simulink model "wlan_phy_tx_pmd"  (Simulink 7.8)
settings: Solver=VariableStepDiscrete  SolverMode=SingleTasking  StartTime=0.0  StopTime=inf  RelTol=1e-3
PostLoadFcn:
  | wlan_phy_tx_init
InitFcn:
  | wlan_phy_tx_init
StartFcn:
  | wlan_phy_tx_init
undefined symbols (not defined in the file): gcbh, ht_preamble_rom, MAX_CP_LEN, MAX_DATA_BITS_PER_SYM_PERIOD, MAX_NCBPS, MAX_NUM_BYTES, MAX_NUM_SC, MAX_NUM_SYMS, mcs_rom_11ag, mcs_rom_11n, Mod_Constellation_16QAM, Mod_Constellation_64QAM, Mod_Constellation_BPSK, Mod_Constellation_QPSK, Preamble_IQ, Preamble_IQ_scaled, tx_sim, wlan_tx_interleave_rom, xlBlockLoadCallback, xlGetNormalizedPeriod
libraries: xbsIndex_r4 x1358, xbsEDKLib_r4 x1
(part 4 of 10)

== system wlan_phy_tx_pmd/IFFT and Cyclic Prefix/Buffer and Cyclic Prefix ==
  note: TODO: Use Sym Cfg values for Cyclic Prefix
      | and Cyclic Shift. Will require buffering through
      | FFT somehow, to keep cfg aligned with corresponding
      | samples. Can't assume upstream logic wil hold cfg
      | constant for duration of IFFT processing...
  I : Inport
  Q : Inport  Port=2
  xkindex : Inport  Port=3
  tvalid : Inport  Port=4
  tlast : Inport  Port=5
  Sym Cfg : Inport  Port=6
  AddSub1 : xbsIndex_r4/AddSub  mode=Addition  use_carryin=off  use_carryout=off  en=off  latency=0  precision=User Defined  arith_type=Unsigned  n_bits=ceil(log2(MAX_NUM_SC))  bin_pt=0  quantization=Truncate  overflow=Wrap  dbl_ovrd=off  use_behavioral_HDL=off  hw_selection=Fabric  pipelined=off  block_type=addsub
  AddSub2 : xbsIndex_r4/AddSub  mode=Subtraction  use_carryin=off  use_carryout=off  en=off  latency=1  precision=Full  arith_type=Unsigned  n_bits=MAX_NUM_SC  bin_pt=14  quantization=Truncate  overflow=Wrap  dbl_ovrd=off  use_behavioral_HDL=off  hw_selection=Fabric  pipelined=off  block_type=addsub
  Constant1 : xbsIndex_r4/Constant  const=0  gui_display_data_type=Fixed-point  arith_type=Unsigned  n_bits=32  bin_pt=0  preci_type=Single  exp_width=8  frac_width=24  explicit_period=off  period=1  equ=P=C  opselect=C  inp2=PCIN>>17  opr=+  inp1=P  carry=CIN  dbl_ovrd=off  block_type=constant
      settings: block_version=VER_STRING_GOES_HERE
  Constant2 : xbsIndex_r4/Constant  const=0  gui_display_data_type=Boolean  arith_type=Boolean  n_bits=1  bin_pt=0  preci_type=Single  exp_width=8  frac_width=24  explicit_period=off  period=1  equ=P=C  opselect=C  inp2=PCIN>>17  opr=+  inp1=P  carry=CIN  dbl_ovrd=off  block_type=constant
      settings: block_version=VER_STRING_GOES_HERE
  Control : Subsystem
  Delay : xbsIndex_r4/Delay  rst=off  infoeditControl=Selection of Reset will increase slice count due to use of real FFs and instead of SRLs  en=off  latency=1  dbl_ovrd=off  reg_retiming=off  block_type=delay
  Delay3 : xbsIndex_r4/Delay  rst=off  infoeditControl=Selection of Reset will increase slice count due to use of real FFs and instead of SRLs  en=off  latency=1  dbl_ovrd=off  reg_retiming=off  block_type=delay
  Dual Port RAM : xbsIndex_r4/Dual Port RAM  depth=MAX_NUM_SC * 1  initVector=0  distributed_mem=Block RAM  init_a=0  init_b=0  rst_a=off  rst_b=off  en_a=off  en_b=off  latency=1  write_mode_A=Read After Write  write_mode_B=Read After Write  dbl_ovrd=off  optimize=Area  block_type=dpram
  Gateway Out{1..8} (8 alike) : xbsIndex_r4/Gateway Out  inherit_from_input=off  hdl_port=off  timing_constraint=None  locs_specified=off  LOCs={}  UseAsDAC=off  DACChannel='1'  block_type=gatewayout
  I/Q Concat : Subsystem
  I/Q Slice : Subsystem
  IFFT Buffer : Scope  NumInputPorts=8
      settings: TimeRange=12000  YMin=0~0~0~0~0~-0.5~-0.5~0  YMax=1~100~1~100~1~0.5~0.5~100
  Terminator : Terminator
  " I" : Outport
  " Q" : Outport  Port=2
  " valid" : Outport  Port=3
  wires:
  I/Q Concat/1(IQ) -> Dual Port RAM/2
  Dual Port RAM/2 -> I/Q Slice/1(IQ)
  I/1 -> I/Q Concat/1(I)
  Q/1 -> I/Q Concat/2(Q)
  xkindex/1 -> Dual Port RAM/1, Gateway Out2/1
  tvalid/1 -> Dual Port RAM/3, Gateway Out1/1
  tlast/1 -> Gateway Out3/1, Control/1(tlast)
  AddSub1/1 -> Dual Port RAM/4, Gateway Out4/1, Delay/1
  [regTx_NUM_SC] -> AddSub2/1
  [regTx_CP_LEN] -> AddSub2/2
  AddSub2/1 -> AddSub1/1
  Constant1/1 -> Dual Port RAM/5
  Constant2/1 -> Dual Port RAM/6
  Dual Port RAM/1 -> Terminator/1
  I/Q Slice/1(I) -> " I"/1, Gateway Out6/1
  I/Q Slice/2(Q) -> " Q"/1, Gateway Out8/1
  Gateway Out1/1 -> IFFT Buffer/1  "IN tvalid"
  Gateway Out2/1 -> IFFT Buffer/2  "IN xkindex"
  Gateway Out3/1 -> IFFT Buffer/3  "IN tlast"
  Gateway Out4/1 -> IFFT Buffer/4  "Rd Addr"
  Gateway Out5/1 -> IFFT Buffer/5  "OUT valid"
  Gateway Out6/1 -> IFFT Buffer/6  "OUT I"
  Gateway Out7/1 -> IFFT Buffer/8  "OUT index"
  Control/2(Valid) -> Delay3/1
  Gateway Out8/1 -> IFFT Buffer/7  "OUT Q"
  Delay/1 -> Gateway Out7/1
  Delay3/1 -> " valid"/1, Gateway Out5/1
  Control/1(Rd Addr) -> AddSub1/2
  Sym Cfg/1 -> ?

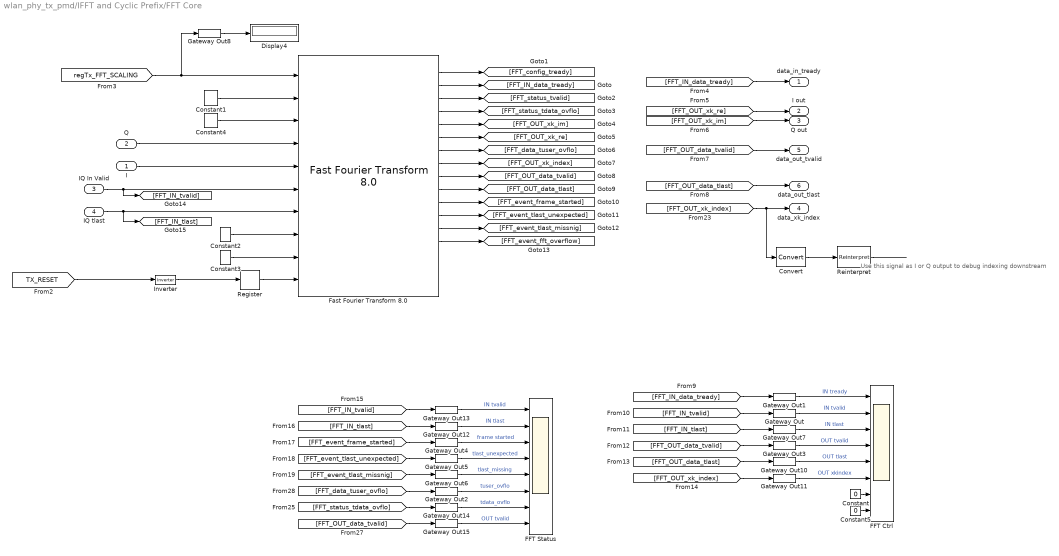
== system wlan_phy_tx_pmd/IFFT and Cyclic Prefix/FFT Core ==
  note: Use this signal as I or Q output
      | to debug indexing downstream
  "I " : Inport
  "Q " : Inport  Port=2
  IQ In Valid : Inport  Port=3
  IQ tlast : Inport  Port=4
  Constant : Constant  Value=0
  Constant1 : xbsIndex_r4/Constant  const=0  gui_display_data_type=Fixed-point  arith_type=Unsigned  n_bits=1  bin_pt=0  preci_type=Single  exp_width=8  frac_width=24  explicit_period=on  period=1  equ=P=C  opselect=C  inp2=PCIN>>17  opr=+  inp1=P  carry=CIN  dbl_ovrd=off  block_type=constant
  Constant2 : xbsIndex_r4/Constant  const=1  gui_display_data_type=Boolean  arith_type=Boolean  n_bits=1  bin_pt=0  preci_type=Single  exp_width=8  frac_width=24  explicit_period=on  period=1  equ=P=C  opselect=C  inp2=PCIN>>17  opr=+  inp1=P  carry=CIN  dbl_ovrd=off  block_type=constant
  Constant3 : xbsIndex_r4/Constant  const=1  gui_display_data_type=Boolean  arith_type=Boolean  n_bits=1  bin_pt=0  preci_type=Single  exp_width=8  frac_width=24  explicit_period=on  period=1  equ=P=C  opselect=C  inp2=PCIN>>17  opr=+  inp1=P  carry=CIN  dbl_ovrd=off  block_type=constant
  Constant4 : xbsIndex_r4/Constant  const=1  gui_display_data_type=Boolean  arith_type=Boolean  n_bits=1  bin_pt=0  preci_type=Single  exp_width=8  frac_width=24  explicit_period=on  period=1  equ=P=C  opselect=C  inp2=PCIN>>17  opr=+  inp1=P  carry=CIN  dbl_ovrd=off  block_type=constant
  Constant5 : Constant  Value=0
  Convert : xbsIndex_r4/Convert  gui_display_data_type=Fixed-point  arith_type="Signed  (2's comp)"  n_bits=16  bin_pt=0  float_type=Single  exp_bits=8  fraction_bits=24  quantization=Truncate  overflow=Wrap  en=off  latency=0  dbl_ovrd=off  pipeline=off  block_type=convert
  Display4 : Display
  FFT Ctrl : Scope  NumInputPorts=8
      settings: TimeRange=4500  YMin=0~0~0~0~0~0~-1~-1  YMax=1~1~1~1~1~80~1~1  SaveName=ScopeData12
  FFT Status : Scope  NumInputPorts=8
      settings: TimeRange=10000  YMin=0~0~0~-1~-1~0~0~0  YMax=1~1~1~1~1~6~6~1  SaveName=ScopeData13
  "Fast Fourier Transform 8.0 " : xbsIndex_r4/Fast Fourier Transform 8.0   transform_length=64  target_clock_frequency=160  target_data_throughput=50  implementation_options=radix_4_burst_io  run_time_configurable_transform_length=off  phase_factor_width=16  scaling_options=scaled  rounding_modes=truncation  aclken=off  aresetn=on  cyclic_prefix_insertion=off  output_ordering=bit_reversed_order  throttle_scheme=nonrealtime  xk_index=on  ovflo=on  trim_axipin_name=on  memory_options_data=block_ram  memory_options_phase_factors=block_ram  number_of_stages_using_block_ram_for_data_and_phase_factors=0  memory_options_reorder=block_ram  memory_options_hybrid=off  complex_mult_type=use_mults_performance  butterfly_type=use_xtremedsp_slices  channels=1  input_ordering=natural_order  input_width=16  ip_name=Fast Fourier Transform  ip_version=8.0  dsptool_ready=true  ipcore_usecache=true  ipcore_useipmodelcache=true  wrapper_available=true  port_translation_map={ 'aclken' => 'en', 'aresetn' => 'rst'}  block_type=xfft_v8_0
  Gateway Out{,1..8,10..15} (15 alike) : xbsIndex_r4/Gateway Out  inherit_from_input=off  hdl_port=off  timing_constraint=None  locs_specified=off  LOCs={}  UseAsDAC=off  DACChannel='1'  block_type=gatewayout
  Inverter : xbsIndex_r4/Inverter  en=off  latency=0  dbl_ovrd=off  block_type=inv
  Register : xbsIndex_r4/Register  init=0  rst=off  en=off  dbl_ovrd=off  block_type=register
  Reinterpret : xbsIndex_r4/Reinterpret  force_arith_type=on  arith_type="Signed  (2's comp)"  force_bin_pt=on  bin_pt=15  block_type=reinterpret
  data_in_tready : Outport
  I out : Outport  Port=2
  Q out : Outport  Port=3
  data_xk_index : Outport  Port=4
  data_out_tvalid : Outport  Port=5
  data_out_tlast : Outport  Port=6
  wires:
  Gateway Out8/1 -> Display4/1
  [regTx_FFT_SCALING] -> Gateway Out8/1, "Fast Fourier Transform 8.0 "/1
  [TX_RESET] -> Inverter/1
  IQ In Valid/1 -> [FFT_IN_tvalid], "Fast Fourier Transform 8.0 "/6
  IQ tlast/1 -> [FFT_IN_tlast], "Fast Fourier Transform 8.0 "/7
  Gateway Out7/1 -> FFT Ctrl/3  "IN tlast"
  Gateway Out6/1 -> FFT Status/5  "tlast_missing"
  Gateway Out5/1 -> FFT Status/4  "tlast_unexpected"
  Gateway Out4/1 -> FFT Status/3  "frame started"
  Gateway Out1/1 -> FFT Ctrl/1  "IN tready"
  Gateway Out/1 -> FFT Ctrl/2  "IN tvalid"
  [FFT_IN_data_tready] -> data_in_tready/1
  [FFT_OUT_xk_re] -> I out/1
  [FFT_OUT_xk_im] -> Q out/1
  [FFT_OUT_data_tvalid] -> data_out_tvalid/1
  [FFT_OUT_data_tlast] -> data_out_tlast/1
  Gateway Out3/1 -> FFT Ctrl/4  "OUT tvalid"
  Gateway Out10/1 -> FFT Ctrl/5  "OUT tlast"
  Gateway Out11/1 -> FFT Ctrl/6  "OUT xkindex"
  Gateway Out12/1 -> FFT Status/2  "IN tlast"
  Gateway Out13/1 -> FFT Status/1  "IN tvalid"
  [FFT_IN_data_tready] -> Gateway Out1/1
  [FFT_IN_tvalid] -> Gateway Out/1
  [FFT_IN_tlast] -> Gateway Out7/1
  [FFT_OUT_data_tvalid] -> Gateway Out3/1
  [FFT_OUT_data_tlast] -> Gateway Out10/1
  [FFT_OUT_xk_index] -> Gateway Out11/1
  [FFT_IN_tvalid] -> Gateway Out13/1
  [FFT_IN_tlast] -> Gateway Out12/1
  [FFT_event_frame_started] -> Gateway Out4/1
  [FFT_event_tlast_unexpected] -> Gateway Out5/1
  [FFT_event_tlast_missnig] -> Gateway Out6/1
  [FFT_OUT_xk_index] -> data_xk_index/1, Convert/1
  Constant/1 -> FFT Ctrl/7
  Constant5/1 -> FFT Ctrl/8
  Gateway Out15/1 -> FFT Status/8  "OUT tvalid"
  [FFT_OUT_data_tvalid] -> Gateway Out15/1
  Constant1/1 -> "Fast Fourier Transform 8.0 "/2
  Constant4/1 -> "Fast Fourier Transform 8.0 "/3
  "Q "/1 -> "Fast Fourier Transform 8.0 "/4
  "I "/1 -> "Fast Fourier Transform 8.0 "/5
  Constant2/1 -> "Fast Fourier Transform 8.0 "/8
  Inverter/1 -> Register/1
  Constant3/1 -> "Fast Fourier Transform 8.0 "/9
  [FFT_data_tuser_ovflo] -> Gateway Out2/1
  Gateway Out2/1 -> FFT Status/6  "tuser_ovflo"
  Gateway Out14/1 -> FFT Status/7  "tdata_ovflo"
  [FFT_status_tdata_ovflo] -> Gateway Out14/1
  "Fast Fourier Transform 8.0 "/1 -> [FFT_config_tready]
  "Fast Fourier Transform 8.0 "/2 -> [FFT_IN_data_tready]
  "Fast Fourier Transform 8.0 "/3 -> [FFT_status_tvalid]
  "Fast Fourier Transform 8.0 "/4 -> [FFT_status_tdata_ovflo]
  "Fast Fourier Transform 8.0 "/5 -> [FFT_OUT_xk_im]
  "Fast Fourier Transform 8.0 "/6 -> [FFT_OUT_xk_re]
  "Fast Fourier Transform 8.0 "/7 -> [FFT_data_tuser_ovflo]
  "Fast Fourier Transform 8.0 "/8 -> [FFT_OUT_xk_index]
  "Fast Fourier Transform 8.0 "/9 -> [FFT_OUT_data_tvalid]
  "Fast Fourier Transform 8.0 "/10 -> [FFT_OUT_data_tlast]
  "Fast Fourier Transform 8.0 "/11 -> [FFT_event_frame_started]
  "Fast Fourier Transform 8.0 "/12 -> [FFT_event_tlast_unexpected]
  "Fast Fourier Transform 8.0 "/13 -> [FFT_event_tlast_missnig]
  "Fast Fourier Transform 8.0 "/14 -> [FFT_event_fft_overflow]
  Convert/1 -> Reinterpret/1
  Reinterpret/1 -> ?
  Register/1 -> "Fast Fourier Transform 8.0 "/10

== system wlan_phy_tx_pmd/IFFT and Cyclic Prefix/FIFO ==
  note: AND not strictly necessary, since FFT
      | only honors tlast when tvalid is asserted.
      | Explicit AND here makes scopes
      | much easier to understand.
  note: This FIFO aids in synchronizing sample generation
      | and feeding the FFT. It would be possible to design
      | the sample buffer control logic not to require
      | this FIFO, but then the logic would need tweaking
      | if the FFT timing or sample processing timing
      | ever change. This FIFO isolates those blocks,
      | at the cost of a little memory
  FFT tready : Inport
  Sym Cfg : Inport  Port=2
  I : Inport  Port=3
  Q : Inport  Port=4
  IQ tvalid : Inport  Port=5
  "IQ tlast " : Inport  Port=6
  AXI FIFO : xbsIndex_r4/AXI FIFO  input_depth_axis=128  actual_fifo_depth_label=130  enable_tdata=on  enable_tdest=off  enable_tstrb=off  enable_tready=on  enable_tid=off  enable_tuser=on  enable_tkeep=off  enable_tlast=on  has_aresetn=on  enable_data_counts_axis=on  fifo_implementation_type_axis=Common Clock Block RAM  trim_axipin_name=on  programmable_full_type_axis=Full  full_threshold_assert_value_axis=0  programmable_empty_type_axis=Empty  empty_threshold_assert_value_axis=1022  block_type=axi_fifo
  Convert : xbsIndex_r4/Convert  gui_display_data_type=Fixed-point  arith_type="Signed  (2's comp)"  n_bits=16  bin_pt=15  float_type=Single  exp_bits=8  fraction_bits=24  quantization=Truncate  overflow=Wrap  en=off  latency=0  dbl_ovrd=off  pipeline=off  block_type=convert
  Convert1 : xbsIndex_r4/Convert  gui_display_data_type=Fixed-point  arith_type="Signed  (2's comp)"  n_bits=16  bin_pt=15  float_type=Single  exp_bits=8  fraction_bits=24  quantization=Truncate  overflow=Wrap  en=off  latency=0  dbl_ovrd=off  pipeline=off  block_type=convert
  FFT IN FIFO : Scope  NumInputPorts=7
      settings: TimeRange=30000  YMin=0~0~0~-0.1~0~-0.1~-0.1  YMax=300~300~1~1.1~4000~1.1~1.1  SaveName=ScopeData20
  FIFO Ctrl : Scope  NumInputPorts=8
      settings: TimeRange=12000  YMin=0~0~0~0~0~0~0~-5  YMax=1~1~5000~1~1~5000~1~5  SaveName=ScopeData21
  Gateway Out{1..15} (15 alike) : xbsIndex_r4/Gateway Out  inherit_from_input=off  hdl_port=off  timing_constraint=None  locs_specified=off  LOCs={}  UseAsDAC=off  DACChannel='1'  block_type=gatewayout
  I/Q Concat : Subsystem
  I/Q Slice : Subsystem
  Inverter : xbsIndex_r4/Inverter  en=off  latency=0  dbl_ovrd=off  block_type=inv
  Logical2 : xbsIndex_r4/Logical  logical_function=AND  inputs=2  en=off  latency=0  precision=Full  arith_type=Unsigned  n_bits=16  bin_pt=0  align_bp=on  dbl_ovrd=off  block_type=logical
  Register : xbsIndex_r4/Register  init=0  rst=off  en=off  dbl_ovrd=off  block_type=register
  " I" : Outport
  " Q" : Outport  Port=2
  " IQ tvalid" : Outport  Port=3
  IQ tlast : Outport  Port=4
  Sym cfg : Outport  Port=5
  FIFO tready : Outport  Port=6
  tag scope: IFFT_FIFO_OCC=global
  wires:
  FFT tready/1 -> Gateway Out8/1, AXI FIFO/2
  IQ tvalid/1 -> AXI FIFO/3, Gateway Out5/1, Gateway Out14/1
  "IQ tlast "/1 -> AXI FIFO/5, Gateway Out6/1, Gateway Out7/1
  I/1 -> Convert/1
  Q/1 -> Convert1/1
  I/Q Concat/1(IQ) -> AXI FIFO/4
  [TX_RESET] -> Inverter/1, Gateway Out13/1
  Inverter/1 -> Register/1
  Convert/1 -> I/Q Concat/1(I)
  Convert1/1 -> I/Q Concat/2(Q)
  Sym Cfg/1 -> AXI FIFO/6, Gateway Out9/1
  AXI FIFO/5 -> FIFO tready/1, Gateway Out4/1
  AXI FIFO/2 -> I/Q Slice/1(IQ)
  AXI FIFO/1 -> " IQ tvalid"/1, Gateway Out1/1, Logical2/1, Gateway Out10/1
  AXI FIFO/3 -> Logical2/2, Gateway Out11/1
  Gateway Out8/1 -> FFT IN FIFO/1  "FFT ready"
  I/Q Slice/1(I) -> " I"/1
  I/Q Slice/2(Q) -> " Q"/1, Gateway Out2/1
  Gateway Out1/1 -> FFT IN FIFO/2  "FIFO out valid"
  Gateway Out2/1 -> FFT IN FIFO/3  "Q out"
  Gateway Out3/1 -> FFT IN FIFO/4  "tlast out"
  Gateway Out4/1 -> FFT IN FIFO/5  "FIFO ready"
  Gateway Out5/1 -> FFT IN FIFO/6  "valid in"
  Gateway Out6/1 -> FFT IN FIFO/7  "tlast in"
  Logical2/1 -> IQ tlast/1, Gateway Out3/1
  AXI FIFO/4 -> Gateway Out12/1, Sym cfg/1
  Gateway Out14/1 -> FIFO Ctrl/1  "VALID In"
  Gateway Out7/1 -> FIFO Ctrl/2  "TLAST In"
  Gateway Out9/1 -> FIFO Ctrl/3  "TUSER In"
  Gateway Out10/1 -> FIFO Ctrl/4  "VALID out"
  Gateway Out11/1 -> FIFO Ctrl/5  "TLAST out"
  Gateway Out12/1 -> FIFO Ctrl/6  "TUSER out"
  Gateway Out13/1 -> FIFO Ctrl/7  "Reset"
  AXI FIFO/6 -> [IFFT_FIFO_OCC], Gateway Out15/1
  Register/1 -> AXI FIFO/1
  Gateway Out15/1 -> FIFO Ctrl/8  "FIFO Occ"

== system wlan_phy_tx_pmd/OFDM Symbol Ctrl/Posedge1 ==
  D : Inport
  Delay : xbsIndex_r4/Delay  rst=off  infoeditControl=Selection of Reset will increase slice count due to use of real FFs and instead of SRLs  en=off  latency=1  dbl_ovrd=off  reg_retiming=off  block_type=delay
      settings: infoedit=Hardware notes: A delay line is a chain, each link of which is an SRL16 followed by a flip-flop. If register retiming is enabled, the delay line is a chain of flip-flops.  xl_area=[1 1 0 0 0 0 0]  block_version=VER_STRING_GOES_HERE
  Inverter : xbsIndex_r4/Inverter  en=off  latency=0  dbl_ovrd=off  block_type=inv
      settings: xl_area=[0 0 0 0 0 0 0]  block_version=VER_STRING_GOES_HERE
  Logical1 : xbsIndex_r4/Logical  logical_function=AND  inputs=2  en=off  latency=0  precision=Full  arith_type=Unsigned  n_bits=8  bin_pt=2  align_bp=on  dbl_ovrd=off  block_type=logical
      settings: xl_area=[1 0 0 1 0 0 0]  block_version=VER_STRING_GOES_HERE
  Q : Outport
  wires:
  Inverter/1 -> Logical1/1
  D/1 -> Logical1/2, Delay/1
  Logical1/1 -> Q/1
  Delay/1 -> Inverter/1

== system wlan_phy_tx_pmd/OFDM Symbol Ctrl/Posedge2 ==
  D : Inport
  Delay : xbsIndex_r4/Delay  rst=off  infoeditControl=Selection of Reset will increase slice count due to use of real FFs and instead of SRLs  en=off  latency=1  dbl_ovrd=off  reg_retiming=off  block_type=delay
      settings: infoedit=Hardware notes: A delay line is a chain, each link of which is an SRL16 followed by a flip-flop. If register retiming is enabled, the delay line is a chain of flip-flops.  xl_area=[1 1 0 0 0 0 0]  block_version=VER_STRING_GOES_HERE
  Inverter : xbsIndex_r4/Inverter  en=off  latency=0  dbl_ovrd=off  block_type=inv
      settings: xl_area=[0 0 0 0 0 0 0]  block_version=VER_STRING_GOES_HERE
  Logical1 : xbsIndex_r4/Logical  logical_function=AND  inputs=2  en=off  latency=0  precision=Full  arith_type=Unsigned  n_bits=8  bin_pt=2  align_bp=on  dbl_ovrd=off  block_type=logical
      settings: xl_area=[1 0 0 1 0 0 0]  block_version=VER_STRING_GOES_HERE
  Q : Outport
  wires:
  Delay/1 -> Inverter/1
  Logical1/1 -> Q/1
  D/1 -> Delay/1, Logical1/2
  Inverter/1 -> Logical1/1

== system wlan_phy_tx_pmd/OFDM Symbol Ctrl/Posedge3 ==
  D : Inport
  Delay : xbsIndex_r4/Delay  rst=off  infoeditControl=Selection of Reset will increase slice count due to use of real FFs and instead of SRLs  en=off  latency=1  dbl_ovrd=off  reg_retiming=off  block_type=delay
      settings: infoedit=Hardware notes: A delay line is a chain, each link of which is an SRL16 followed by a flip-flop. If register retiming is enabled, the delay line is a chain of flip-flops.  xl_area=[1 1 0 0 0 0 0]  block_version=VER_STRING_GOES_HERE
  Inverter : xbsIndex_r4/Inverter  en=off  latency=0  dbl_ovrd=off  block_type=inv
      settings: xl_area=[0 0 0 0 0 0 0]  block_version=VER_STRING_GOES_HERE
  Logical1 : xbsIndex_r4/Logical  logical_function=AND  inputs=2  en=off  latency=0  precision=Full  arith_type=Unsigned  n_bits=8  bin_pt=2  align_bp=on  dbl_ovrd=off  block_type=logical
      settings: xl_area=[1 0 0 1 0 0 0]  block_version=VER_STRING_GOES_HERE
  Q : Outport
  wires:
  Delay/1 -> Inverter/1
  Logical1/1 -> Q/1
  D/1 -> Delay/1, Logical1/2
  Inverter/1 -> Logical1/1

== system wlan_phy_tx_pmd/OFDM Symbol Ctrl/S-R Latch1 ==
  S : Inport
  R : Inport  Port=2
  Constant1 : xbsIndex_r4/Constant  const=1  gui_display_data_type=Fixed-point  arith_type=Boolean  n_bits=1  bin_pt=0  preci_type=Single  exp_width=8  frac_width=24  explicit_period=off  period=1  equ=P=C  opselect=C  inp2=PCIN>>17  opr=+  inp1=P  carry=CIN  dbl_ovrd=off  block_type=constant
      settings: block_version=VER_STRING_GOES_HERE
  Convert1 : xbsIndex_r4/Convert  gui_display_data_type=Boolean  arith_type=Boolean  n_bits=1  bin_pt=0  float_type=Single  exp_bits=8  fraction_bits=24  quantization=Truncate  overflow=Wrap  en=off  latency=0  dbl_ovrd=off  pipeline=off  block_type=convert
  Convert2 : xbsIndex_r4/Convert  gui_display_data_type=Boolean  arith_type=Boolean  n_bits=1  bin_pt=0  float_type=Single  exp_bits=8  fraction_bits=24  quantization=Truncate  overflow=Wrap  en=off  latency=0  dbl_ovrd=off  pipeline=off  block_type=convert
  Register2 : xbsIndex_r4/Register  init=0  rst=on  en=on  dbl_ovrd=off  block_type=register
      settings: xl_area=[1 1 0 0 0 0 0]  block_version=VER_STRING_GOES_HERE
  Q : Outport
  wires:
  Convert2/1 -> Register2/3
  Convert1/1 -> Register2/2
  Constant1/1 -> Register2/1
  R/1 -> Convert1/1
  Register2/1 -> Q/1
  S/1 -> Convert2/1

== system wlan_phy_tx_pmd/OFDM Symbol Ctrl/S-R Latch2 ==
  S : Inport
  R : Inport  Port=2
  Constant1 : xbsIndex_r4/Constant  const=1  gui_display_data_type=Fixed-point  arith_type=Boolean  n_bits=1  bin_pt=0  preci_type=Single  exp_width=8  frac_width=24  explicit_period=off  period=1  equ=P=C  opselect=C  inp2=PCIN>>17  opr=+  inp1=P  carry=CIN  dbl_ovrd=off  block_type=constant
      settings: block_version=VER_STRING_GOES_HERE
  Convert1 : xbsIndex_r4/Convert  gui_display_data_type=Boolean  arith_type=Boolean  n_bits=1  bin_pt=0  float_type=Single  exp_bits=8  fraction_bits=24  quantization=Truncate  overflow=Wrap  en=off  latency=0  dbl_ovrd=off  pipeline=off  block_type=convert
  Convert2 : xbsIndex_r4/Convert  gui_display_data_type=Boolean  arith_type=Boolean  n_bits=1  bin_pt=0  float_type=Single  exp_bits=8  fraction_bits=24  quantization=Truncate  overflow=Wrap  en=off  latency=0  dbl_ovrd=off  pipeline=off  block_type=convert
  Register2 : xbsIndex_r4/Register  init=0  rst=on  en=on  dbl_ovrd=off  block_type=register
      settings: xl_area=[1 1 0 0 0 0 0]  block_version=VER_STRING_GOES_HERE
  Q : Outport
  wires:
  S/1 -> Convert2/1
  Register2/1 -> Q/1
  R/1 -> Convert1/1
  Constant1/1 -> Register2/1
  Convert1/1 -> Register2/2
  Convert2/1 -> Register2/3

== system wlan_phy_tx_pmd/OFDM Symbol Ctrl/S-R Latch3 ==
  S : Inport
  R : Inport  Port=2
  Constant1 : xbsIndex_r4/Constant  const=1  gui_display_data_type=Fixed-point  arith_type=Boolean  n_bits=1  bin_pt=0  preci_type=Single  exp_width=8  frac_width=24  explicit_period=off  period=1  equ=P=C  opselect=C  inp2=PCIN>>17  opr=+  inp1=P  carry=CIN  dbl_ovrd=off  block_type=constant
      settings: block_version=VER_STRING_GOES_HERE
  Convert1 : xbsIndex_r4/Convert  gui_display_data_type=Boolean  arith_type=Boolean  n_bits=1  bin_pt=0  float_type=Single  exp_bits=8  fraction_bits=24  quantization=Truncate  overflow=Wrap  en=off  latency=0  dbl_ovrd=off  pipeline=off  block_type=convert
  Convert2 : xbsIndex_r4/Convert  gui_display_data_type=Boolean  arith_type=Boolean  n_bits=1  bin_pt=0  float_type=Single  exp_bits=8  fraction_bits=24  quantization=Truncate  overflow=Wrap  en=off  latency=0  dbl_ovrd=off  pipeline=off  block_type=convert
  Register2 : xbsIndex_r4/Register  init=0  rst=on  en=on  dbl_ovrd=off  block_type=register
      settings: xl_area=[1 1 0 0 0 0 0]  block_version=VER_STRING_GOES_HERE
  Q : Outport
  wires:
  S/1 -> Convert2/1
  Register2/1 -> Q/1
  R/1 -> Convert1/1
  Constant1/1 -> Register2/1
  Convert1/1 -> Register2/2
  Convert2/1 -> Register2/3

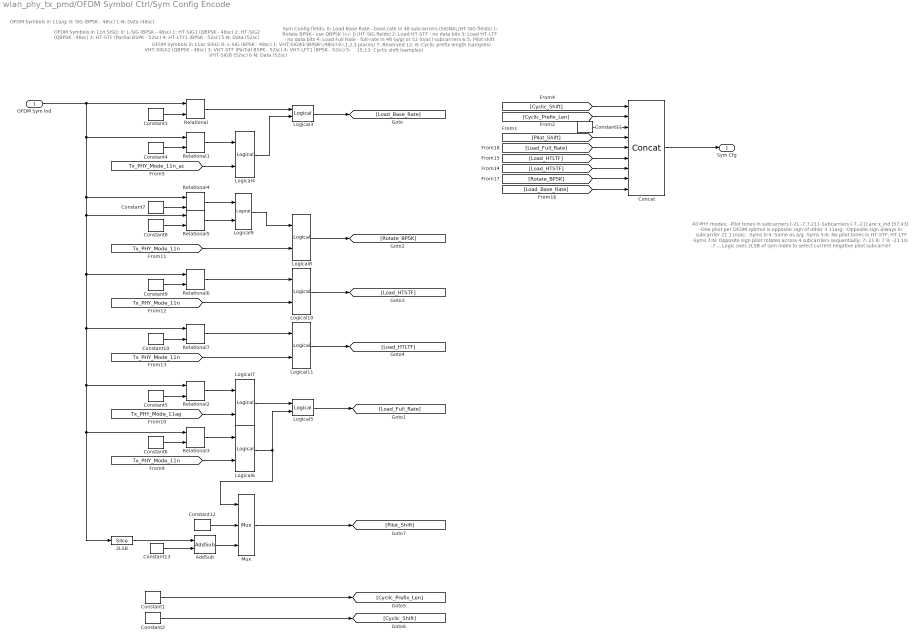
== system wlan_phy_tx_pmd/OFDM Symbol Ctrl/Sym Config Encode ==
  note: Sym Config fields:
      |   0: Load Base Rate - base-rate in 48 subcarriers (SIGNAL/HT-SIG fields)
      |   1: Rotate BPSK - use QBPSK (+/- j) (HT-SIG fields)
      |   2: Load HT-STF - no data bits
      |   3: Load HT-LTF - no data bits
      |   4: Load Full Rate - full-rate in 48 (a/g) or 52 (n/ac) subcarriers
      | 6:5: Pilot shift (Rotate negative pilot 0,1,2,3 places)
      |   7: Reserved
      |
      | 12: 8: Cyclic prefix length (samples)
      | 15:13: Cyclic shift (samples)
  note: OFDM Symbols in 11ac SISO:
      | 0: L-SIG (BPSK - 48sc)
      | 1: VHT-SIGA1 (BPSK - 48sc)
      | 2: VHT-SIGA2 (QBPSK - 48sc)
      | 3: VHT-STF (Partial BSPK - 52sc)
      | 4: VHT-LFT1 (BPSK - 52sc)
      | 5: VHT-SIGB (52sc)
      | 6-N: Data (52sc)
  note: OFDM Symbols in 11n SISO:
      | 0: L-SIG (BPSK - 48sc)
      | 1: HT-SIG1 (QBPSK - 48sc)
      | 2: HT-SIG2 (QBPSK - 48sc)
      | 3: HT-STF (Partial BSPK - 52sc)
      | 4: HT-LTF1 (BPSK - 52sc)
      | 5-N: Data (52sc)
  note: OFDM Symbols in 11a/g:
      | 0: SIG (BPSK - 48sc)
      | 1-N: Data (48sc)
  note: All PHY modes:
      | -Pilot tones in subcarriers [-21,-7,7,21]
      | -Subcarriers [-7,-21] are x_ind [57,43]
      | -One pilot per OFDM sybmol is opposite sign of other 3
      |
      | 11a/g:
      | -Opposite sign always in subcarrier 21
      |
      | 11n/ac:
      | -Syms 0:4: Same as a/g
      | -Syms 5:6: No pilot tones in HT-STF, HT-LTF
      | -Syms 7:N: Opposite sign pilot rotates across 4 subcarriers sequentially:
      |    7: 21
      |    8: 7
      |    9: -21
      |    10: -7
      |     ...
      | Logic uses 2LSB of sym index to select current negative pilot subcarrier
  OFDM Sym Ind : Inport
  2LSB : xbsIndex_r4/Slice  nbits=2  boolean_output=off  mode=Lower Bit Location + Width  bit1=0  base1=MSB of Input  bit0=0  base0=LSB of Input  dbl_ovrd=off  block_type=slice
  AddSub : xbsIndex_r4/AddSub  mode=Addition  use_carryin=off  use_carryout=off  en=off  latency=0  precision=User Defined  arith_type=Unsigned  n_bits=2  bin_pt=0  quantization=Truncate  overflow=Wrap  dbl_ovrd=off  use_behavioral_HDL=off  hw_selection=Fabric  pipelined=off  block_type=addsub
  Concat : xbsIndex_r4/Concat  num_inputs=9  dbl_ovrd=off  block_type=concat
  Constant1 : xbsIndex_r4/Constant  const=16  gui_display_data_type=Fixed-point  arith_type=Unsigned  n_bits=5  bin_pt=0  preci_type=Single  exp_width=8  frac_width=24  explicit_period=on  period=1  equ=P=C  opselect=C  inp2=PCIN>>17  opr=+  inp1=P  carry=CIN  dbl_ovrd=off  block_type=constant
  Constant10 : xbsIndex_r4/Constant  const=4  gui_display_data_type=Fixed-point  arith_type=Unsigned  n_bits=3  bin_pt=0  preci_type=Single  exp_width=8  frac_width=24  explicit_period=off  period=1  equ=P=C  opselect=C  inp2=PCIN>>17  opr=+  inp1=P  carry=CIN  dbl_ovrd=off  block_type=constant
  Constant11 : xbsIndex_r4/Constant  const=0  gui_display_data_type=Fixed-point  arith_type=Unsigned  n_bits=1  bin_pt=0  preci_type=Single  exp_width=8  frac_width=24  explicit_period=off  period=1  equ=P=C  opselect=C  inp2=PCIN>>17  opr=+  inp1=P  carry=CIN  dbl_ovrd=off  block_type=constant
  Constant12 : xbsIndex_r4/Constant  const=0  gui_display_data_type=Fixed-point  arith_type=Unsigned  n_bits=2  bin_pt=0  preci_type=Single  exp_width=8  frac_width=24  explicit_period=off  period=1  equ=P=C  opselect=C  inp2=PCIN>>17  opr=+  inp1=P  carry=CIN  dbl_ovrd=off  block_type=constant
  Constant13 : xbsIndex_r4/Constant  const=3  gui_display_data_type=Fixed-point  arith_type=Unsigned  n_bits=2  bin_pt=0  preci_type=Single  exp_width=8  frac_width=24  explicit_period=off  period=8  equ=P=C  opselect=C  inp2=PCIN>>17  opr=+  inp1=P  carry=CIN  dbl_ovrd=off  block_type=constant
  Constant2 : xbsIndex_r4/Constant  const=0  gui_display_data_type=Fixed-point  arith_type=Unsigned  n_bits=5  bin_pt=0  preci_type=Single  exp_width=8  frac_width=24  explicit_period=on  period=1  equ=P=C  opselect=C  inp2=PCIN>>17  opr=+  inp1=P  carry=CIN  dbl_ovrd=off  block_type=constant
  Constant3 : xbsIndex_r4/Constant  const=0  gui_display_data_type=Fixed-point  arith_type=Unsigned  n_bits=1  bin_pt=0  preci_type=Single  exp_width=8  frac_width=24  explicit_period=off  period=1  equ=P=C  opselect=C  inp2=PCIN>>17  opr=+  inp1=P  carry=CIN  dbl_ovrd=off  block_type=constant
  Constant4 : xbsIndex_r4/Constant  const=2  gui_display_data_type=Fixed-point  arith_type=Unsigned  n_bits=2  bin_pt=0  preci_type=Single  exp_width=8  frac_width=24  explicit_period=off  period=1  equ=P=C  opselect=C  inp2=PCIN>>17  opr=+  inp1=P  carry=CIN  dbl_ovrd=off  block_type=constant
  Constant5 : xbsIndex_r4/Constant  const=1  gui_display_data_type=Fixed-point  arith_type=Unsigned  n_bits=1  bin_pt=0  preci_type=Single  exp_width=8  frac_width=24  explicit_period=off  period=1  equ=P=C  opselect=C  inp2=PCIN>>17  opr=+  inp1=P  carry=CIN  dbl_ovrd=off  block_type=constant
  Constant6 : xbsIndex_r4/Constant  const=5  gui_display_data_type=Fixed-point  arith_type=Unsigned  n_bits=3  bin_pt=0  preci_type=Single  exp_width=8  frac_width=24  explicit_period=off  period=1  equ=P=C  opselect=C  inp2=PCIN>>17  opr=+  inp1=P  carry=CIN  dbl_ovrd=off  block_type=constant
  Constant7 : xbsIndex_r4/Constant  const=1  gui_display_data_type=Fixed-point  arith_type=Unsigned  n_bits=1  bin_pt=0  preci_type=Single  exp_width=8  frac_width=24  explicit_period=off  period=1  equ=P=C  opselect=C  inp2=PCIN>>17  opr=+  inp1=P  carry=CIN  dbl_ovrd=off  block_type=constant
  Constant8 : xbsIndex_r4/Constant  const=2  gui_display_data_type=Fixed-point  arith_type=Unsigned  n_bits=2  bin_pt=0  preci_type=Single  exp_width=8  frac_width=24  explicit_period=off  period=1  equ=P=C  opselect=C  inp2=PCIN>>17  opr=+  inp1=P  carry=CIN  dbl_ovrd=off  block_type=constant
  Constant9 : xbsIndex_r4/Constant  const=3  gui_display_data_type=Fixed-point  arith_type=Unsigned  n_bits=2  bin_pt=0  preci_type=Single  exp_width=8  frac_width=24  explicit_period=off  period=1  equ=P=C  opselect=C  inp2=PCIN>>17  opr=+  inp1=P  carry=CIN  dbl_ovrd=off  block_type=constant
  Logical{4,6..8,10..11} (6 alike) : xbsIndex_r4/Logical  logical_function=AND  inputs=2  en=off  latency=0  precision=Full  arith_type=Unsigned  n_bits=8  bin_pt=2  align_bp=on  dbl_ovrd=off  block_type=logical
      settings: xl_area=[1 0 0 1 0 0 0]  block_version=VER_STRING_GOES_HERE
  Logical3 : xbsIndex_r4/Logical  logical_function=OR  inputs=2  en=off  latency=0  precision=Full  arith_type=Unsigned  n_bits=8  bin_pt=2  align_bp=on  dbl_ovrd=off  block_type=logical
      settings: xl_area=[1 0 0 1 0 0 0]  block_version=VER_STRING_GOES_HERE
  Logical5 : xbsIndex_r4/Logical  logical_function=OR  inputs=2  en=off  latency=0  precision=Full  arith_type=Unsigned  n_bits=8  bin_pt=2  align_bp=on  dbl_ovrd=off  block_type=logical
      settings: xl_area=[1 0 0 1 0 0 0]  block_version=VER_STRING_GOES_HERE
  Logical9 : xbsIndex_r4/Logical  logical_function=OR  inputs=2  en=off  latency=0  precision=Full  arith_type=Unsigned  n_bits=8  bin_pt=2  align_bp=on  dbl_ovrd=off  block_type=logical
      settings: xl_area=[1 0 0 1 0 0 0]  block_version=VER_STRING_GOES_HERE
  Mux : xbsIndex_r4/Mux  inputs=2  en=off  latency=0  precision=Full  arith_type=Unsigned  n_bits=16  bin_pt=14  quantization=Truncate  overflow=Wrap  dbl_ovrd=off  block_type=mux
  Relational{,4..7} (5 alike) : xbsIndex_r4/Relational  mode=a=b  en=off  latency=0  dbl_ovrd=off  block_type=relational
  Relational1 : xbsIndex_r4/Relational  mode=a<=b  en=off  latency=0  dbl_ovrd=off  block_type=relational
  Relational2 : xbsIndex_r4/Relational  mode=a>=b  en=off  latency=0  dbl_ovrd=off  block_type=relational
  Relational3 : xbsIndex_r4/Relational  mode=a>=b  en=off  latency=0  dbl_ovrd=off  block_type=relational
  Sym Cfg : Outport
  wires:
  Constant3/1 -> Relational/2
  Relational/1 -> Logical3/1
  [Tx_PHY_Mode_11n_ac] -> Logical4/2
  Relational1/1 -> Logical4/1
  Constant4/1 -> Relational1/2
  Logical4/1 -> Logical3/2
  Constant5/1 -> Relational2/2
  [Tx_PHY_Mode_11n] -> Logical6/2
  Relational3/1 -> Logical6/1
  Constant6/1 -> Relational3/2
  Logical6/1 -> Logical5/2, Mux/1
  Logical5/1 -> [Load_Full_Rate]
  Logical7/1 -> Logical5/1
  Relational2/1 -> Logical7/1
  [Tx_PHY_Mode_11ag] -> Logical7/2
  [Tx_PHY_Mode_11n] -> Logical8/2
  Constant7/1 -> Relational4/2
  Constant8/1 -> Relational5/2
  Relational4/1 -> Logical9/1
  Relational5/1 -> Logical9/2
  Logical9/1 -> Logical8/1
  Logical8/1 -> [Rotate_BPSK]
  [Tx_PHY_Mode_11n] -> Logical10/2
  Constant9/1 -> Relational6/2
  Relational6/1 -> Logical10/1
  Logical10/1 -> [Load_HTSTF]
  [Tx_PHY_Mode_11n] -> Logical11/2
  Constant10/1 -> Relational7/2
  Relational7/1 -> Logical11/1
  Logical11/1 -> [Load_HTLTF]
  OFDM Sym Ind/1 -> Relational/1, Relational1/1, Relational5/1, Relational6/1, Relational7/1, Relational2/1, Relational3/1, 2LSB/1, Relational4/1
  [Load_Full_Rate] -> Concat/5
  [Load_HTLTF] -> Concat/6
  [Load_HTSTF] -> Concat/7
  [Rotate_BPSK] -> Concat/8
  [Load_Base_Rate] -> Concat/9
  Constant1/1 -> [Cyclic_Prefix_Len]
  Constant2/1 -> [Cyclic_Shift]
  Constant11/1 -> Concat/3
  [Cyclic_Prefix_Len] -> Concat/2
  [Cyclic_Shift] -> Concat/1
  Concat/1 -> Sym Cfg/1
  Logical3/1 -> [Load_Base_Rate]
  2LSB/1 -> AddSub/1
  [Pilot_Shift] -> Concat/4
  Constant12/1 -> Mux/2
  Mux/1 -> [Pilot_Shift]
  AddSub/1 -> Mux/3
  Constant13/1 -> AddSub/2

== system wlan_phy_tx_pmd/OFDM Symbol Ctrl/Sym Counter ==
  note: Use SR latch to skip counter increment
      | on first sym (indexes syms by 0)
  Start Sym : Inport
  Delay : xbsIndex_r4/Delay  rst=off  infoeditControl=Selection of Reset will increase slice count due to use of real FFs and instead of SRLs  en=off  latency=1  dbl_ovrd=off  reg_retiming=off  block_type=delay
  Logical2 : xbsIndex_r4/Logical  logical_function=AND  inputs=2  en=off  latency=0  precision=Full  arith_type=Unsigned  n_bits=8  bin_pt=2  align_bp=on  dbl_ovrd=off  block_type=logical
      settings: xl_area=[1 0 0 1 0 0 0]  block_version=VER_STRING_GOES_HERE
  S-R Latch1 : Subsystem
  Sym Counter : xbsIndex_r4/Counter  cnt_type=Free Running  cnt_to=47  operation=Up  start_count=0  cnt_by_val=1  arith_type=Unsigned  n_bits=ceil(log2(MAX_NUM_SYMS))  bin_pt=0  load_pin=off  rst=on  en=on  explicit_period=off  period=1  dbl_ovrd=off  use_behavioral_HDL=off  implementation=Fabric  block_type=counter
  Sym Ind : Outport
  " Start Sym" : Outport  Port=2
  wires:
  [TX_RESET] -> Sym Counter/1
  Logical2/1 -> Sym Counter/2
  S-R Latch1/1(Q) -> Logical2/2
  [TX_RESET] -> S-R Latch1/2(R)
  Start Sym/1 -> Logical2/1, S-R Latch1/1(S), Delay/1
  Sym Counter/1 -> Sym Ind/1
  Delay/1 -> " Start Sym"/1

== system wlan_phy_tx_pmd/OFDM Symbol Ctrl/Sym Samp Counter ==
  Sym Started : Inport
  Sym Cfg : Inport  Port=2
  AddSub : xbsIndex_r4/AddSub  mode=Addition  use_carryin=off  use_carryout=off  en=on  latency=1  precision=Full  arith_type=Unsigned  n_bits=16  bin_pt=14  quantization=Truncate  overflow=Wrap  dbl_ovrd=off  use_behavioral_HDL=off  hw_selection=Fabric  pipelined=off  block_type=addsub
  Inverter : xbsIndex_r4/Inverter  en=off  latency=0  dbl_ovrd=off  block_type=inv
  Logical : xbsIndex_r4/Logical  logical_function=AND  inputs=2  en=off  latency=0  precision=Full  arith_type=Unsigned  n_bits=16  bin_pt=0  align_bp=on  dbl_ovrd=off  block_type=logical
  Logical1 : xbsIndex_r4/Logical  logical_function=OR  inputs=2  en=off  latency=0  precision=Full  arith_type=Unsigned  n_bits=16  bin_pt=0  align_bp=on  dbl_ovrd=off  block_type=logical
  Logical2 : xbsIndex_r4/Logical  logical_function=OR  inputs=2  en=off  latency=0  precision=Full  arith_type=Unsigned  n_bits=16  bin_pt=0  align_bp=on  dbl_ovrd=off  block_type=logical
  MCode : xbsIndex_r4/MCode  mfname=sym_config_decode  explicit_period=on  period=1  inputsTable={'boundInpExpr'=>[''],'inputs'=>['sym_cfg']}  outputsTable={'outputs'=>['load_base_rate','rotate_bpsk','load_htstf','load_htltf','load_full_rate','pilot_shift','cyclic_prefix','cyclic_shift'],'suppressOut'=>['off','off','off','off','off','off','off','off']}  dbl_ovrd=off  enable_stdout=off  enable_debug=off  suppress_output=on  defparams={}  hide_port_list={}  block_type=mcode
  Posedge1 : Subsystem
  Posedge2 : Subsystem
  Relational2 : xbsIndex_r4/Relational  mode=a>=b  en=off  latency=0  dbl_ovrd=off  block_type=relational
  S-R Latch2 : Subsystem
  Samp Counter : xbsIndex_r4/Counter  cnt_type=Free Running  cnt_to=47  operation=Up  start_count=0  cnt_by_val=1  arith_type=Unsigned  n_bits=ceil(log2(MAX_NUM_SYMS))  bin_pt=0  load_pin=off  rst=on  en=on  explicit_period=off  period=1  dbl_ovrd=off  use_behavioral_HDL=off  implementation=Fabric  block_type=counter
  Start Next : Outport
  wires:
  Logical/1 -> Samp Counter/2
  [regTx_NUM_SC] -> AddSub/1
  Sym Cfg/1 -> MCode/1
  Samp Counter/1 -> Relational2/1
  MCode/7 -> AddSub/2
  Sym Started/1 -> Posedge1/1(D)
  Posedge1/1(Q) -> S-R Latch2/1(S)
  S-R Latch2/1(Q) -> Logical/1, Inverter/1
  [TX_IQ_SAMP_CE] -> Logical/2
  Relational2/1 -> Posedge2/1(D)
  AddSub/1 -> Relational2/2
  Posedge2/1(Q) -> Start Next/1, Logical1/2
  Logical1/1 -> S-R Latch2/2(R)
  Logical2/1 -> Samp Counter/1
  Inverter/1 -> Logical2/2
  [TX_RESET] -> Logical2/1, Logical1/1, AddSub/3

== system wlan_phy_tx_pmd/PSDU Syms Gen/Convolutional Encoder ==
  Sym Cfg : Inport
  Tx Bit : Inport  Port=2
  Tx Bit tvalid : Inport  Port=3
  Tx Bit tlast : Inport  Port=4
  A XOR : xbsIndex_r4/Logical  logical_function=XOR  inputs=5  en=on  latency=1  precision=Full  arith_type=Unsigned  n_bits=8  bin_pt=2  align_bp=on  dbl_ovrd=off  block_type=logical
      settings: xl_area=[0, 0, 0, 0, 0, 0, 0]  block_version=VER_STRING_GOES_HERE
  B XOR : xbsIndex_r4/Logical  logical_function=XOR  inputs=5  en=on  latency=1  precision=Full  arith_type=Unsigned  n_bits=8  bin_pt=2  align_bp=on  dbl_ovrd=off  block_type=logical
      settings: xl_area=[0, 0, 0, 0, 0, 0, 0]  block_version=VER_STRING_GOES_HERE
  Concat : xbsIndex_r4/Concat  num_inputs=2  dbl_ovrd=off  block_type=concat
  Convert : xbsIndex_r4/Convert  gui_display_data_type=Boolean  arith_type=Boolean  n_bits=16  bin_pt=14  float_type=Single  exp_bits=8  fraction_bits=24  quantization=Truncate  overflow=Wrap  en=off  latency=0  dbl_ovrd=off  pipeline=off  block_type=convert
  Convert2 : xbsIndex_r4/Convert  gui_display_data_type=Boolean  arith_type=Boolean  n_bits=16  bin_pt=14  float_type=Single  exp_bits=8  fraction_bits=24  quantization=Truncate  overflow=Wrap  en=off  latency=0  dbl_ovrd=off  pipeline=off  block_type=convert
  Delay1 : xbsIndex_r4/Delay  rst=off  infoeditControl=Selection of Reset will increase slice count due to use of real FFs and instead of SRLs  en=off  latency=1  dbl_ovrd=off  reg_retiming=off  block_type=delay
  Delay2 : xbsIndex_r4/Delay  rst=off  infoeditControl=Selection of Reset will increase slice count due to use of real FFs and instead of SRLs  en=off  latency=1  dbl_ovrd=off  reg_retiming=off  block_type=delay
  Delay3 : xbsIndex_r4/Delay  rst=off  infoeditControl=Selection of Reset will increase slice count due to use of real FFs and instead of SRLs  en=off  latency=1  dbl_ovrd=off  reg_retiming=off  block_type=delay
  Gateway Out1 : xbsIndex_r4/Gateway Out  inherit_from_input=off  hdl_port=off  timing_constraint=None  locs_specified=off  LOCs={}  UseAsDAC=off  DACChannel='1'  block_type=gatewayout
  Gateway Out4 : xbsIndex_r4/Gateway Out  inherit_from_input=off  hdl_port=off  timing_constraint=None  locs_specified=off  LOCs={}  UseAsDAC=off  DACChannel='1'  block_type=gatewayout
  Register{,1..5} (6 alike) : xbsIndex_r4/Register  init=0  rst=on  en=on  dbl_ovrd=off  block_type=register
      settings: xl_area=[0, 0, 0, 0, 0, 0, 0]  block_version=VER_STRING_GOES_HERE
  To Workspace : ToWorkspace  VariableName=tx_coded_bits  SampleTime=-1  SaveFormat=Array
  To Workspace1 : ToWorkspace  VariableName=tx_coded_bits_vld  SampleTime=-1  SaveFormat=Array
  " Sym Cfg" : Outport
  Enc Bit A : Outport  Port=2
  Enc Bit B : Outport  Port=3
  Enc Bits tvalid : Outport  Port=4
  Enc Bits tlast : Outport  Port=5
  wires:
  Tx Bit tvalid/1 -> Convert2/1
  [TX_RESET] -> Convert/1
  B XOR/1 -> Enc Bit B/1, Concat/1
  A XOR/1 -> Enc Bit A/1, Concat/2
  Register5/1 -> B XOR/5, A XOR/5
  Tx Bit/1 -> B XOR/1, A XOR/1, Register/1
  Register4/1 -> A XOR/4, Register5/1
  Register3/1 -> Register4/1
  Register2/1 -> B XOR/4, A XOR/3, Register3/1
  Register1/1 -> B XOR/3, A XOR/2, Register2/1
  Register/1 -> B XOR/2, Register1/1
  Convert/1 -> Register/2, Register1/2, Register2/2, Register3/2, Register5/2, Register4/2
  Convert2/1 -> B XOR/6, A XOR/6, Register/3, Register1/3, Register2/3, Register3/3, Register4/3, Register5/3, Delay3/1
  Delay3/1 -> Enc Bits tvalid/1, Gateway Out1/1
  Sym Cfg/1 -> Delay1/1
  Delay1/1 -> " Sym Cfg"/1
  Tx Bit tlast/1 -> Delay2/1
  Delay2/1 -> Enc Bits tlast/1
  Concat/1 -> Gateway Out4/1
  Gateway Out4/1 -> To Workspace/1
  Gateway Out1/1 -> To Workspace1/1

== system wlan_phy_tx_pmd/PSDU Syms Gen/Index Gen ==
  Sym Cfg : Inport
  Start Sym : Inport  Port=2
  Bit Index Gen : Subsystem
  Bits Per Sym : Subsystem
  MCode : xbsIndex_r4/MCode  mfname=sym_config_decode  explicit_period=on  period=1  inputsTable={'boundInpExpr'=>[''],'inputs'=>['sym_cfg']}  outputsTable={'outputs'=>['load_base_rate','rotate_bpsk','load_htstf','load_htltf','load_full_rate','pilot_shift','cyclic_prefix','cyclic_shift'],'suppressOut'=>['off','off','off','off','off','off','off','off']}  dbl_ovrd=off  enable_stdout=off  enable_debug=off  suppress_output=on  defparams={}  hide_port_list={}  block_type=mcode
  " Sym Cfg" : Outport
  Byte Ind : Outport  Port=2
  Byte Ind Valid : Outport  Port=3
  Bit Sel : Outport  Port=4
  Bit Sel Valid : Outport  Port=5
  wires:
  MCode/5 -> Bits Per Sym/3(Full Rate)
  Sym Cfg/1 -> " Sym Cfg"/1, MCode/1
  Start Sym/1 -> Bits Per Sym/1(Start)
  Bits Per Sym/1(Rd En) -> Bit Index Gen/1(Bit Rd En)
  MCode/1 -> Bits Per Sym/2(Base Rate)
  Bit Index Gen/1(Byte Ind) -> Byte Ind/1
  Bit Index Gen/3(Bit Sel) -> Bit Sel/1
  Bit Index Gen/4(Bit Sel Valid) -> Bit Sel Valid/1
  Bit Index Gen/2(Byte Ind Valid) -> Byte Ind Valid/1

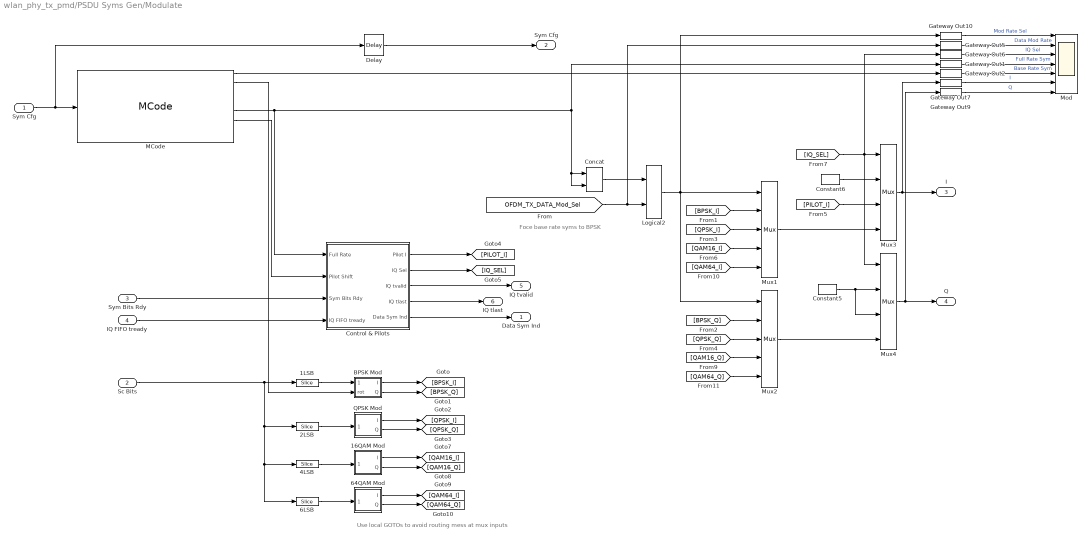
== system wlan_phy_tx_pmd/PSDU Syms Gen/Modulate ==
  note: Foce base rate syms to BPSK
  note: Use local GOTOs to avoid
      | routing mess at mux inputs
  Sym Cfg : Inport
  Sc Bits : Inport  Port=2
  Sym Bits Rdy : Inport  Port=3
  IQ FIFO tready : Inport  Port=4
  16QAM Mod : Subsystem
  1LSB : xbsIndex_r4/Slice  nbits=1  boolean_output=off  mode=Lower Bit Location + Width  bit1=0  base1=MSB of Input  bit0=0  base0=LSB of Input  dbl_ovrd=off  block_type=slice
  2LSB : xbsIndex_r4/Slice  nbits=2  boolean_output=off  mode=Lower Bit Location + Width  bit1=0  base1=MSB of Input  bit0=0  base0=LSB of Input  dbl_ovrd=off  block_type=slice
  4LSB : xbsIndex_r4/Slice  nbits=4  boolean_output=off  mode=Lower Bit Location + Width  bit1=0  base1=MSB of Input  bit0=0  base0=LSB of Input  dbl_ovrd=off  block_type=slice
  64QAM Mod : Subsystem
  6LSB : xbsIndex_r4/Slice  nbits=6  boolean_output=off  mode=Lower Bit Location + Width  bit1=0  base1=MSB of Input  bit0=0  base0=LSB of Input  dbl_ovrd=off  block_type=slice
  BPSK Mod : Subsystem
  Concat : xbsIndex_r4/Concat  num_inputs=2  dbl_ovrd=off  block_type=concat
  Constant5 : xbsIndex_r4/Constant  const=0  gui_display_data_type=Fixed-point  arith_type=Signed (2's comp)  n_bits=12  bin_pt=11  preci_type=Single  exp_width=8  frac_width=24  explicit_period=off  period=1  equ=P=C  opselect=C  inp2=PCIN>>17  opr=+  inp1=P  carry=CIN  dbl_ovrd=off  block_type=constant
  Constant6 : xbsIndex_r4/Constant  const=0  gui_display_data_type=Fixed-point  arith_type=Signed (2's comp)  n_bits=12  bin_pt=11  preci_type=Single  exp_width=8  frac_width=24  explicit_period=off  period=1  equ=P=C  opselect=C  inp2=PCIN>>17  opr=+  inp1=P  carry=CIN  dbl_ovrd=off  block_type=constant
  Control & Pilots : Subsystem
  Delay : xbsIndex_r4/Delay  rst=off  infoeditControl=Selection of Reset will increase slice count due to use of real FFs and instead of SRLs  en=off  latency=1  dbl_ovrd=off  reg_retiming=off  block_type=delay
  Gateway Out{1..2,5..7,9..10} (7 alike) : xbsIndex_r4/Gateway Out  inherit_from_input=off  hdl_port=off  timing_constraint=None  locs_specified=off  LOCs={}  UseAsDAC=off  DACChannel='1'  block_type=gatewayout
  Logical2 : xbsIndex_r4/Logical  logical_function=AND  inputs=2  en=off  latency=0  precision=Full  arith_type=Unsigned  n_bits=16  bin_pt=0  align_bp=on  dbl_ovrd=off  block_type=logical
  MCode : xbsIndex_r4/MCode  mfname=sym_config_decode  explicit_period=on  period=1  inputsTable={'boundInpExpr'=>[''],'inputs'=>['sym_cfg']}  outputsTable={'outputs'=>['load_base_rate','rotate_bpsk','load_htstf','load_htltf','load_full_rate','pilot_shift','cyclic_prefix','cyclic_shift'],'suppressOut'=>['off','off','off','off','off','off','off','off']}  dbl_ovrd=off  enable_stdout=off  enable_debug=off  suppress_output=on  defparams={}  hide_port_list={}  block_type=mcode
  "Mod " : Scope  NumInputPorts=7
      settings: TimeRange=10000  YMin=0~0~0~-2~0~-0.1~-0.1  YMax=300~300~1~2~4000~1.1~1.1  SaveName=ScopeData28
  Mux1 : xbsIndex_r4/Mux  inputs=4  en=off  latency=0  precision=Full  arith_type=Unsigned  n_bits=16  bin_pt=14  quantization=Truncate  overflow=Wrap  dbl_ovrd=off  block_type=mux
  Mux2 : xbsIndex_r4/Mux  inputs=4  en=off  latency=0  precision=Full  arith_type=Unsigned  n_bits=16  bin_pt=14  quantization=Truncate  overflow=Wrap  dbl_ovrd=off  block_type=mux
  Mux3 : xbsIndex_r4/Mux  inputs=3  en=off  latency=0  precision=Full  arith_type=Unsigned  n_bits=16  bin_pt=14  quantization=Truncate  overflow=Wrap  dbl_ovrd=off  block_type=mux
  Mux4 : xbsIndex_r4/Mux  inputs=3  en=off  latency=0  precision=Full  arith_type=Unsigned  n_bits=16  bin_pt=14  quantization=Truncate  overflow=Wrap  dbl_ovrd=off  block_type=mux
  QPSK Mod : Subsystem
  Data Sym Ind : Outport
  " Sym Cfg" : Outport  Port=2
  I : Outport  Port=3
  Q : Outport  Port=4
  IQ tvalid : Outport  Port=5
  IQ tlast : Outport  Port=6
  wires:
  [QAM64_I] -> Mux1/5
  [QAM64_Q] -> Mux2/5
  BPSK Mod/1(I) -> [BPSK_I]
  BPSK Mod/2(Q) -> [BPSK_Q]
  QPSK Mod/1(I) -> [QPSK_I]
  QPSK Mod/2(Q) -> [QPSK_Q]
  [BPSK_Q] -> Mux2/2
  [BPSK_I] -> Mux1/2
  [QPSK_Q] -> Mux2/3
  Logical2/1 -> Mux1/1, Mux2/1, Gateway Out10/1
  [QPSK_I] -> Mux1/3
  Constant5/1 -> Mux4/2, Mux4/3
  Constant6/1 -> Mux3/2
  [PILOT_I] -> Mux3/3
  Mux1/1 -> Mux3/4
  Mux2/1 -> Mux4/4
  Mux3/1 -> I/1, Gateway Out7/1
  Mux4/1 -> Q/1, Gateway Out9/1
  [IQ_SEL] -> Mux3/1, Mux4/1, Gateway Out6/1
  Gateway Out10/1 -> "Mod "/1  "Mod Rate Sel"
  Gateway Out5/1 -> "Mod "/2  "Data Mod Rate"
  Gateway Out6/1 -> "Mod "/3  "IQ Sel"
  Gateway Out7/1 -> "Mod "/6  "I"
  Gateway Out9/1 -> "Mod "/7  "Q"
  16QAM Mod/1(I) -> [QAM16_I]
  16QAM Mod/2(Q) -> [QAM16_Q]
  [QAM16_I] -> Mux1/4
  [QAM16_Q] -> Mux2/4
  64QAM Mod/1(I) -> [QAM64_I]
  64QAM Mod/2(Q) -> [QAM64_Q]
  Sc Bits/1 -> 4LSB/1, 6LSB/1, 2LSB/1, 1LSB/1
  Control & Pilots/1(Pilot I) -> [PILOT_I]
  Control & Pilots/2(IQ Sel) -> [IQ_SEL]
  Sym Bits Rdy/1 -> Control & Pilots/3(Sym Bits Rdy)
  Sym Cfg/1 -> Delay/1, MCode/1
  [OFDM_TX_DATA_Mod_Sel] -> Logical2/2, Gateway Out5/1
  Control & Pilots/3(IQ tvalid) -> IQ tvalid/1
  Control & Pilots/4(IQ tlast) -> IQ tlast/1
  Control & Pilots/5(Data Sym Ind) -> Data Sym Ind/1
  Delay/1 -> " Sym Cfg"/1
  IQ FIFO tready/1 -> Control & Pilots/4(IQ FIFO tready)
  1LSB/1 -> BPSK Mod/1(b[0])
  2LSB/1 -> QPSK Mod/1(b[1:0])
  4LSB/1 -> 16QAM Mod/1(b[3:0])
  6LSB/1 -> 64QAM Mod/1(b[5:0])
  Concat/1 -> Logical2/1
  MCode/5 -> Control & Pilots/1(Full Rate), Concat/1, Concat/2, Gateway Out1/1
  Gateway Out1/1 -> "Mod "/4  "Full Rate Sym"
  Gateway Out2/1 -> "Mod "/5  "Base Rate Sym"
  MCode/1 -> Gateway Out2/1
  MCode/2 -> BPSK Mod/2(rot)
  MCode/6 -> Control & Pilots/2(Pilot Shift)
